simulink model "untitled"  (R2019a)
settings: Solver=VariableStepAuto  StartTime=0.0  StopTime=1  RelTol=1e-3
settings Model: Creator=Sayeed  LastModifiedBy=Sayeed

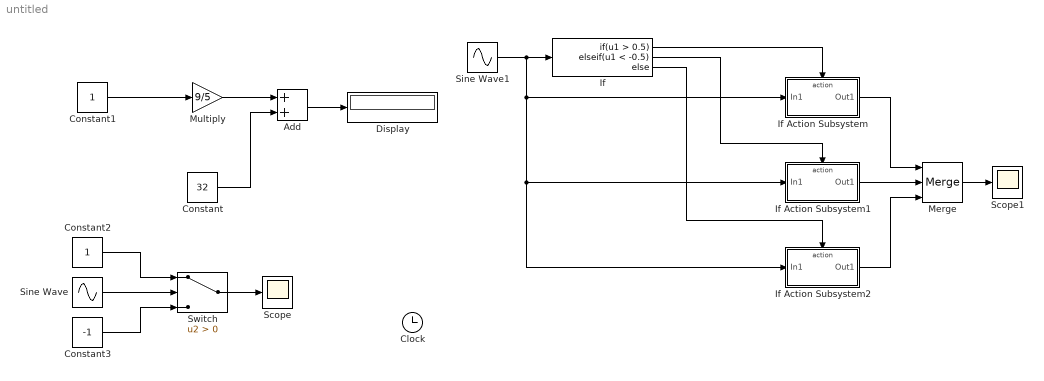
== system untitled ==
  Add : Sum
  Clock : Clock
  Constant : Constant  Value=32
  Constant1 : Constant
  Constant2 : Constant
  Constant3 : Constant  Value=-1
  Display : Display
  If : If  IfExpression=u1 > 0.5  ElseIfExpressions=u1 < -0.5
  If Action Subsystem : Subsystem  TreatAsAtomicUnit=on
  If Action Subsystem1 : Subsystem  TreatAsAtomicUnit=on
  If Action Subsystem2 : Subsystem  TreatAsAtomicUnit=on
  Merge : Merge  Inputs=3
  Multiply : Gain  Gain=9/5
  Scope : Scope
  Scope1 : Scope
  Sine Wave : Sin  Frequency=10  SampleTime=0
  Sine Wave1 : Sin  Frequency=10  SampleTime=0
  Switch : Switch  Criteria=u2 > Threshold
  wires:
  Multiply/1 -> Add/1
  Constant/1 -> Add/2
  Add/1 -> Display/1
  Constant1/1 -> Multiply/1
  Sine Wave/1 -> Switch/2
  Constant2/1 -> Switch/1
  Constant3/1 -> Switch/3
  Switch/1 -> Scope/1
  If/1 -> If Action Subsystem/Action
  If/2 -> If Action Subsystem1/Action
  If/3 -> If Action Subsystem2/Action
  Sine Wave1/1 -> If Action Subsystem/1(In1), If Action Subsystem1/1(In1), If Action Subsystem2/1(In1), If/1
  If Action Subsystem1/1(Out1) -> Merge/2
  If Action Subsystem/1(Out1) -> Merge/1
  If Action Subsystem2/1(Out1) -> Merge/3
  Merge/1 -> Scope1/1

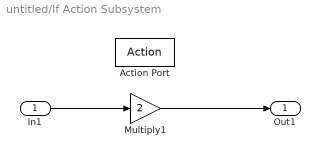
== system untitled/If Action Subsystem ==
  In1 : Inport
  Action Port : ActionPort  ActionPortLabel=if(u1 > 0.5)
  Multiply1 : Gain  Gain=2
  Out1 : Outport
  wires:
  In1/1 -> Multiply1/1
  Multiply1/1 -> Out1/1

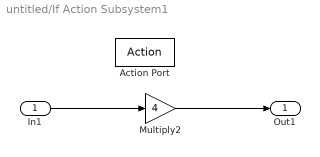
== system untitled/If Action Subsystem1 ==
  In1 : Inport
  Action Port : ActionPort  ActionPortLabel=elseif(u1 < -0.5)
  Multiply2 : Gain  Gain=4
  Out1 : Outport
  wires:
  In1/1 -> Multiply2/1
  Multiply2/1 -> Out1/1

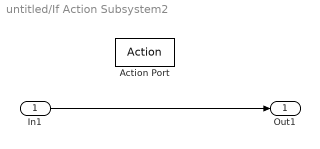
== system untitled/If Action Subsystem2 ==
  In1 : Inport
  Action Port : ActionPort  ActionPortLabel=else
  Out1 : Outport
  wires:
  In1/1 -> Out1/1
